simulink model "arlht_elhossini"  (R2020a)
settings: Solver=FixedStepDiscrete  StartTime=0.0  StopTime=inf  RelTol=1e-3
InitFcn:
  | % Clear workspace
  | clc; clear; close all;
  | 
  | fs = 250e6;
  | 
  | % Set parameters
  | height = 600;
  | width = 800;
  | sobelThreshold = 30;
  | dTheta = 180/16;
  | theta = (0:dTheta:180-dTheta);
  | 
  | % Derive variables
  | maxRho = ceil(sqrt((height/2)^2+(width/2)^2));
  | nRho = maxRho*2;
  | nTheta = length(theta);
  | 
  | % Read in image and resize
  | I = imread('chess.jpg');
  | Ir = imresize(I, [height, width]);
  | 
  | % Get greyscale
  | Y = rgb2gray(Ir);
  | 
  | % Get Sobel and Gradient
  | [edge, dir, mag] = SobelEdge(Y, 100);
  | dirNew = floor(dir/dTheta)*dTheta;
  | simDirNew = dirNew*4;
  | simDirNew(edge==0) = 255*4;
  | 
  | % Create input array
  | inarray = uint16(simDirNew);
StopFcn:
  | [hps, Aopt, rbm] = ARLHT(edge, dirNew, dTheta, 1, 0, 4);
  | plot3DHPS(hps);
  | 
  | simHps = reshape(out.simout, [nRho, nTheta]);
  | plot3DHPS(simHps);
values from neighbouring files (symbols this model uses):
  dir = rad2deg(atan(Gy./Gx))    [SobelEdge.m]
libraries: simulink x39, hdlsllib x26, library x3, dspsrcs4 x1
(part 1 of 2)
settings Model: DataTypeOverride=Off  SimulationMode=rapid-accelerator  Creator=david  LastModifiedBy=david
settings OptimizationCC: BlockReduction=off  ConditionallyExecuteInputs=off  DefaultParameterBehavior=Inlined
settings DebuggingCC: AlgebraicLoopMsg=error  SingleTaskRateTransMsg=error
settings HardwareCC: ProdBitPerPointer=32  ProdBitPerSizeT=32  ProdBitPerPtrDiffT=32  ProdLargestAtomicFloat=None  ProdIntDivRoundTo=Undefined  ProdEndianess=Unspecified  ProdWordSize=32  ProdHWDeviceType=ASIC/FPGA->ASIC/FPGA  TargetBitPerPointer=64  TargetBitPerSizeT=64  TargetBitPerPtrDiffT=64  TargetLongLongMode=on  TargetIntDivRoundTo=Zero  TargetEndianess=LittleEndian  TargetWordSize=64  TargetHWDeviceType=Custom Processor->MATLAB Host Computer  ProdEqTarget=off

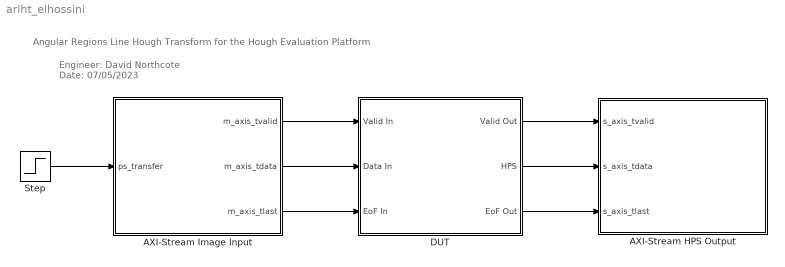
== system arlht_elhossini ==
  note: Angular Regions Line Hough Transform for the Hough Evaluation Platform
  note: Engineer: David Northcote
      | Date: 07/05/2023
  AXI-Stream HPS Output : Subsystem  mask{height=nRho, width=nTheta, clk=1/fs, d=0}
      mask prompts: height "Image Height:"; width "Image Width:"; clk "Clock Rate:"; d "Frame Capture Number"
      mask DialogControl DescGroupVar Prompt: AXI-Stream Image Output
      mask DialogControl DescTextVar Prompt: Image output using the AXI-Stream interface. Simulates an AXI DMA write channel.
      mask DialogControl ParameterGroupVar Prompt: Main
  AXI-Stream Image Input : Subsystem  mask{image=inarray, clk=1/fs}
      mask prompts: image "Input Image:"; clk "Clock Rate:"
      mask init:
      | [height, width] = size(image);
      mask DialogControl DescGroupVar Prompt: AXI-Stream Image Input
      mask DialogControl DescTextVar Prompt: This block simulates an AXI-Stream image input for interfacing to a hardware accelerator or IP Core.
      mask DialogControl ParameterGroupVar Prompt: Main
  DUT : Subsystem  TreatAsAtomicUnit=on
  Step : Step  Time=2/150e6  SampleTime=1/fs
  wires:
  AXI-Stream Image Input/1(m_axis_tvalid) -> DUT/1(Valid In)
  AXI-Stream Image Input/2(m_axis_tdata) -> DUT/2(Data In)
  AXI-Stream Image Input/3(m_axis_tlast) -> DUT/3(EoF In)
  DUT/1(Valid Out) -> AXI-Stream HPS Output/1(s_axis_tvalid)
  DUT/2(HPS) -> AXI-Stream HPS Output/2(s_axis_tdata)
  DUT/3(EoF Out) -> AXI-Stream HPS Output/3(s_axis_tlast)
  Step/1 -> AXI-Stream Image Input/1(ps_transfer)

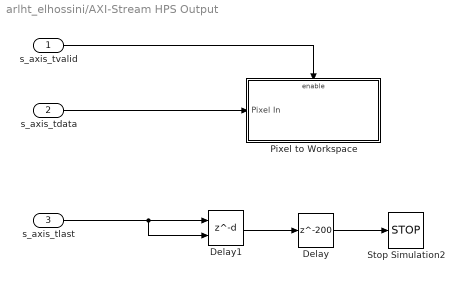
== system arlht_elhossini/AXI-Stream HPS Output ==
  s_axis_tvalid : Inport
  s_axis_tdata : Inport  Port=2
  s_axis_tlast : Inport  Port=3
  Delay : Delay  DelayLength=200
  Delay1 : Delay  DelayLength=d  ShowEnablePort=on
      settings: InputPortMap=u0,e6
  Pixel to Workspace : Subsystem
  Stop Simulation2 : Stop
  wires:
  s_axis_tvalid/1 -> Pixel to Workspace/Enable
  s_axis_tdata/1 -> Pixel to Workspace/1(Pixel In)
  s_axis_tlast/1 -> Delay1/2, Delay1/1
  Delay1/1 -> Delay/1
  Delay/1 -> Stop Simulation2/1

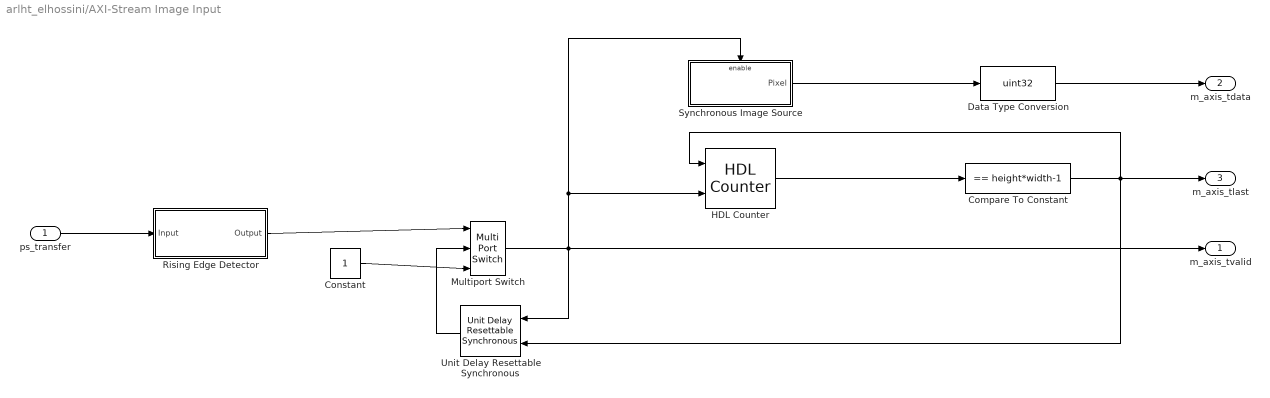
== system arlht_elhossini/AXI-Stream Image Input ==
  ps_transfer : Inport
  Compare To Constant : simulink/Logic and Bit Operations/Compare To Constant  relop===  const=height*width-1  OutDataTypeStr=boolean
  Constant : Constant  OutDataTypeStr=boolean  SampleTime=-1
  Data Type Conversion : DataTypeConversion  OutDataTypeStr=uint32
  HDL Counter : hdlsllib/Sources/HDL Counter  CountType=Free running  CountInit=0  CountStep=1  CountMax=width*height-1  CountFromType=Initial value  CountFrom=0  CountResetPort=on  CountLoadPort=off  CountEnbPort=on  CountDirPort=off  CountDataType=Unsigned  CountWordLen=32  CountFracLen=0  CountSampTime=1
  Multiport Switch : MultiPortSwitch  DataPortOrder=Zero-based contiguous  Inputs=2  zeroidx=on
  Rising Edge Detector : Subsystem
  Synchronous Image Source : Subsystem
  Unit Delay Resettable Synchronous : hdlsllib/Discrete/Unit Delay Resettable Synchronous  InitialCondition=0.0  SampleTime=-1
      settings: SourceProductBaseCode=SL
  m_axis_tvalid : Outport
  m_axis_tdata : Outport  Port=2
  m_axis_tlast : Outport  Port=3
  wires:
  HDL Counter/1 -> Compare To Constant/1
  Synchronous Image Source/1(Pixel) -> Data Type Conversion/1
  Multiport Switch/1 -> Unit Delay Resettable Synchronous/1, HDL Counter/2, Synchronous Image Source/Enable, m_axis_tvalid/1
  Compare To Constant/1 -> Unit Delay Resettable Synchronous/2, HDL Counter/1, m_axis_tlast/1
  Data Type Conversion/1 -> m_axis_tdata/1
  ps_transfer/1 -> Rising Edge Detector/1(Input)
  Unit Delay Resettable Synchronous/1 -> Multiport Switch/2
  Rising Edge Detector/1(Output) -> Multiport Switch/1
  Constant/1 -> Multiport Switch/3

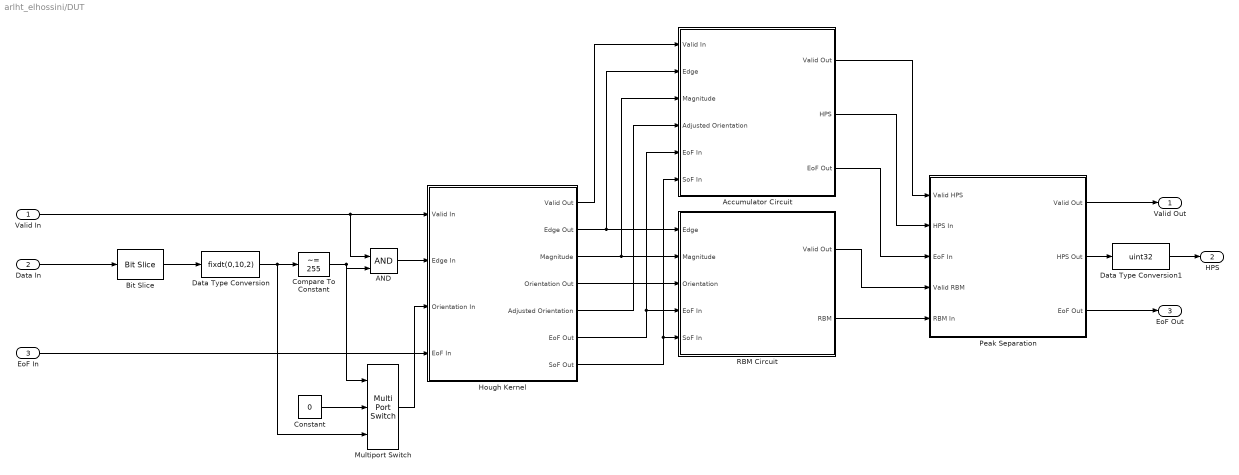
== system arlht_elhossini/DUT ==
  Valid In : Inport
  Data In : Inport  Port=2
  EoF In : Inport  Port=3
  AND : Logic  IconShape=distinctive  AllPortsSameDT=off  OutDataTypeStr=boolean
  Accumulator Circuit : Subsystem  AncestorBlock=library/Accumulator Circuit  mask{height=height, width=width, rhoBits=ceil(log2(maxRho*2*4)), nTheta=nTheta, nRho=nRho}
      mask prompts: height "Image Height:"; width "Image Width:"; rhoBits "Address Bits:"; nTheta "Number Theta:"; nRho "Number Rho:"
      mask init:
      | kTheta = 4;
  Bit Slice : hdlsllib/Logic and Bit Operations/Bit Slice  lidx=9  ridx=0
      settings: SourceProductBaseCode=SL
  Compare To Constant : simulink/Logic and Bit Operations/Compare To Constant  relop=~=  const=255  OutDataTypeStr=boolean
  Constant : Constant  Value=0  OutDataTypeStr=Inherit: Inherit via back propagation  SampleTime=-1
  Data Type Conversion : DataTypeConversion  OutDataTypeStr=fixdt(0,10,2)  ConvertRealWorld=Stored Integer (SI)
  Data Type Conversion1 : DataTypeConversion  OutDataTypeStr=uint32
  Hough Kernel : Subsystem  AncestorBlock=library/Hough Kernel  mask{rhoBits=ceil(log2(maxRho*2)), height=height, width=width, dTheta=dTheta}
      mask prompts: rhoBits "Address Bits:"; height "Image Height:"; width "Image Width:"; dTheta "Theta Resolution:"
      mask init:
      | kTheta = 4;
      | maxRho = ceil(sqrt((height/2)^2+(width/2)^2));
      | theta = (0:dTheta:180-dTheta);
      | gamma = (theta(end) + dTheta)/kTheta;
  Multiport Switch : MultiPortSwitch  DataPortOrder=Zero-based contiguous  Inputs=2  zeroidx=on
  Peak Separation : Subsystem  AncestorBlock=library/Peak Separation  mask{nRho=nRho, nTheta=nTheta}
      mask prompts: nRho "HPS Height:"; nTheta "HPS Width:"
      mask DialogControl DescGroupVar Prompt: Peak Separation
      mask DialogControl ParameterGroupVar Prompt: Main
  RBM Circuit : Subsystem  AncestorBlock=library/RBM Circuit  mask{height=height, width=width, nTheta=nTheta, rhoBits=ceil(log2(maxRho*2)), nRho=nRho}
      mask prompts: height "Image Height:"; width "Image Width:"; nTheta "Number Theta:"; rhoBits "Address Bits:"; nRho "Number Rho:"
  Valid Out : Outport  VectorParamsAs1DForOutWhenUnconnected=off
  HPS : Outport  Port=2  VectorParamsAs1DForOutWhenUnconnected=off
  EoF Out : Outport  Port=3  VectorParamsAs1DForOutWhenUnconnected=off
  wires:
  Accumulator Circuit/2(HPS) -> Peak Separation/2(HPS In)
  Hough Kernel/4(Orientation Out) -> RBM Circuit/3(Orientation)
  Hough Kernel/1(Valid Out) -> Accumulator Circuit/1(Valid In)
  Hough Kernel/3(Magnitude) -> Accumulator Circuit/3(Magnitude), RBM Circuit/2(Magnitude)
  EoF In/1 -> Hough Kernel/4(EoF In)
  RBM Circuit/2(RBM) -> Peak Separation/5(RBM In)
  Hough Kernel/5(Adjusted Orientation) -> Accumulator Circuit/4(Adjusted Orientation)
  Hough Kernel/2(Edge Out) -> Accumulator Circuit/2(Edge), RBM Circuit/1(Edge)
  Hough Kernel/6(EoF Out) -> Accumulator Circuit/5(EoF In), RBM Circuit/4(EoF In)
  Hough Kernel/7(SoF Out) -> Accumulator Circuit/6(SoF In), RBM Circuit/5(SoF In)
  Peak Separation/2(HPS Out) -> Data Type Conversion1/1
  Peak Separation/3(EoF Out) -> EoF Out/1
  RBM Circuit/1(Valid Out) -> Peak Separation/4(Valid RBM)
  Peak Separation/1(Valid Out) -> Valid Out/1
  Accumulator Circuit/1(Valid Out) -> Peak Separation/1(Valid HPS)
  Accumulator Circuit/3(EoF Out) -> Peak Separation/3(EoF In)
  Multiport Switch/1 -> Hough Kernel/3(Orientation In)
  Constant/1 -> Multiport Switch/2
  Data In/1 -> Bit Slice/1
  Data Type Conversion/1 -> Multiport Switch/3, Compare To Constant/1
  AND/1 -> Hough Kernel/2(Edge In)
  Compare To Constant/1 -> AND/2, Multiport Switch/1
  Valid In/1 -> AND/1, Hough Kernel/1(Valid In)
  Data Type Conversion1/1 -> HPS/1
  Bit Slice/1 -> Data Type Conversion/1

== system arlht_elhossini/AXI-Stream HPS Output/Pixel to Workspace ==
  Pixel In : Inport
  Enable : EnablePort
  To Workspace : ToWorkspace  VariableName=simout  SampleTime=-1
      settings: MaxDataPoints=height*width  Save2DSignal=2-D array (concatenate along first dimension)
  wires:
  Pixel In/1 -> To Workspace/1

== system arlht_elhossini/AXI-Stream Image Input/Rising Edge Detector ==
  Input : Inport
  AND : Logic  IconShape=distinctive  AllPortsSameDT=off  OutDataTypeStr=boolean
  Delay : Delay  DelayLength=1
  NOT : Logic  Operator=NOT  IconShape=distinctive  AllPortsSameDT=off  OutDataTypeStr=boolean
  Output : Outport  VectorParamsAs1DForOutWhenUnconnected=off
  wires:
  NOT/1 -> Delay/1
  Input/1 -> AND/2, NOT/1
  Delay/1 -> AND/1
  AND/1 -> Output/1

== system arlht_elhossini/AXI-Stream Image Input/Synchronous Image Source ==
  Enable : EnablePort
  Signal From Workspace : dspsrcs4/Signal From Workspace  X=reshape(image', [height*width, 1])  Ts=clk  nsamps=1  OutputAfterFinalValue=Cyclic repetition  ignoreOrWarnInputAndFrameLengths=off  OutputFrames=off
  Pixel : Outport
  wires:
  Signal From Workspace/1 -> Pixel/1

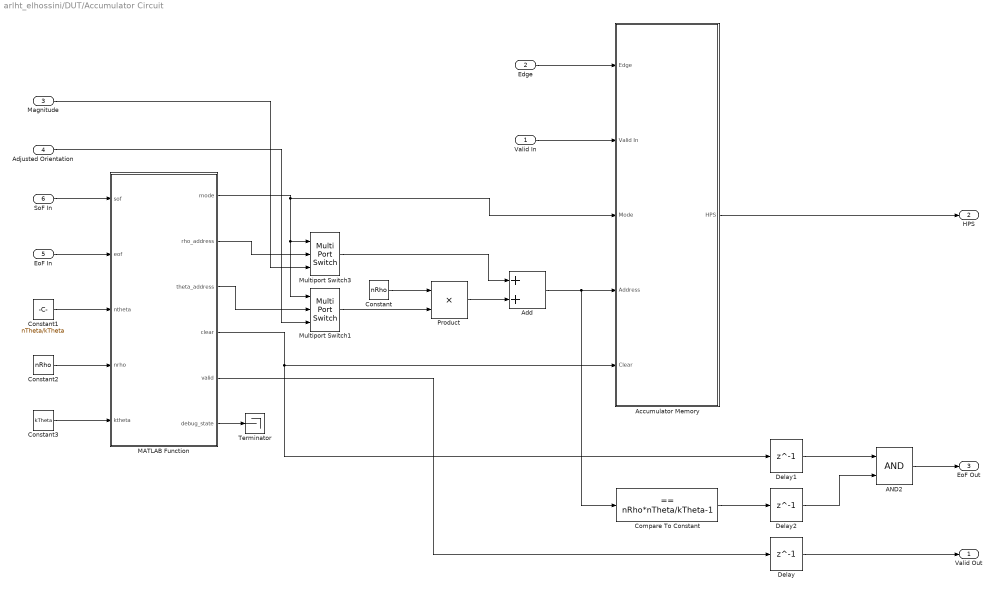
== system arlht_elhossini/DUT/Accumulator Circuit ==
  Valid In : Inport
  Edge : Inport  Port=2
  Magnitude : Inport  Port=3
  Adjusted Orientation : Inport  Port=4
  EoF In : Inport  Port=5
  SoF In : Inport  Port=6
  AND2 : Logic  IconShape=distinctive  AllPortsSameDT=off  OutDataTypeStr=boolean
  Accumulator Memory : Subsystem
  Add : Sum  OutDataTypeStr=fixdt(0,ceil(log2(nRho*nTheta/kTheta)),0)
  Compare To Constant : simulink/Logic and Bit Operations/Compare To Constant  relop===  const=nRho*nTheta/kTheta-1  OutDataTypeStr=boolean
  Constant : Constant  Value=nRho  OutDataTypeStr=fixdt(0,ceil(log2(nRho+1)),0)  SampleTime=-1
  Constant1 : Constant  Value=nTheta/kTheta  OutDataTypeStr=uint8  SampleTime=-1
  Constant2 : Constant  Value=nRho  OutDataTypeStr=uint16  SampleTime=-1
  Constant3 : Constant  Value=kTheta  OutDataTypeStr=uint8  SampleTime=-1
  Delay : Delay  DelayLength=1  InitialCondition=0  UseCircularBuffer=on
  Delay1 : Delay  DelayLength=1  InitialCondition=0  UseCircularBuffer=on
  Delay2 : Delay  DelayLength=1  InitialCondition=0  UseCircularBuffer=on
  MATLAB Function : MATLAB Function  TreatAsAtomicUnit=on
  Multiport Switch1 : MultiPortSwitch  DataPortOrder=Zero-based contiguous  Inputs=2  zeroidx=on
  Multiport Switch3 : MultiPortSwitch  DataPortOrder=Zero-based contiguous  Inputs=2  zeroidx=on
  Product : Product  OutDataTypeStr=fixdt(0,ceil(log2(nRho*(nTheta/kTheta-1))),0)
  Terminator : Terminator
  Valid Out : Outport
  HPS : Outport  Port=2
  EoF Out : Outport  Port=3
  wires:
  MATLAB Function/6(debug_state) -> Terminator/1
  SoF In/1 -> MATLAB Function/1(sof)
  MATLAB Function/4(clear) -> Delay1/1, Accumulator Memory/5(Clear)
  MATLAB Function/5(valid) -> Delay/1
  Delay/1 -> Valid Out/1
  AND2/1 -> EoF Out/1
  Delay1/1 -> AND2/1
  Delay2/1 -> AND2/2
  Constant1/1 -> MATLAB Function/3(ntheta)
  Constant2/1 -> MATLAB Function/4(nrho)
  Constant3/1 -> MATLAB Function/5(ktheta)
  Compare To Constant/1 -> Delay2/1
  Magnitude/1 -> Multiport Switch3/3
  Adjusted Orientation/1 -> Multiport Switch1/3
  Edge/1 -> Accumulator Memory/1(Edge)
  Valid In/1 -> Accumulator Memory/2(Valid In)
  Accumulator Memory/1(HPS) -> HPS/1
  Add/1 -> Compare To Constant/1, Accumulator Memory/4(Address)
  Multiport Switch1/1 -> Product/2
  Multiport Switch3/1 -> Add/1
  Product/1 -> Add/2
  Constant/1 -> Product/1
  MATLAB Function/1(mode) -> Multiport Switch1/1, Multiport Switch3/1, Accumulator Memory/3(Mode)
  MATLAB Function/2(rho_address) -> Multiport Switch3/2
  MATLAB Function/3(theta_address) -> Multiport Switch1/2
  EoF In/1 -> MATLAB Function/2(eof)

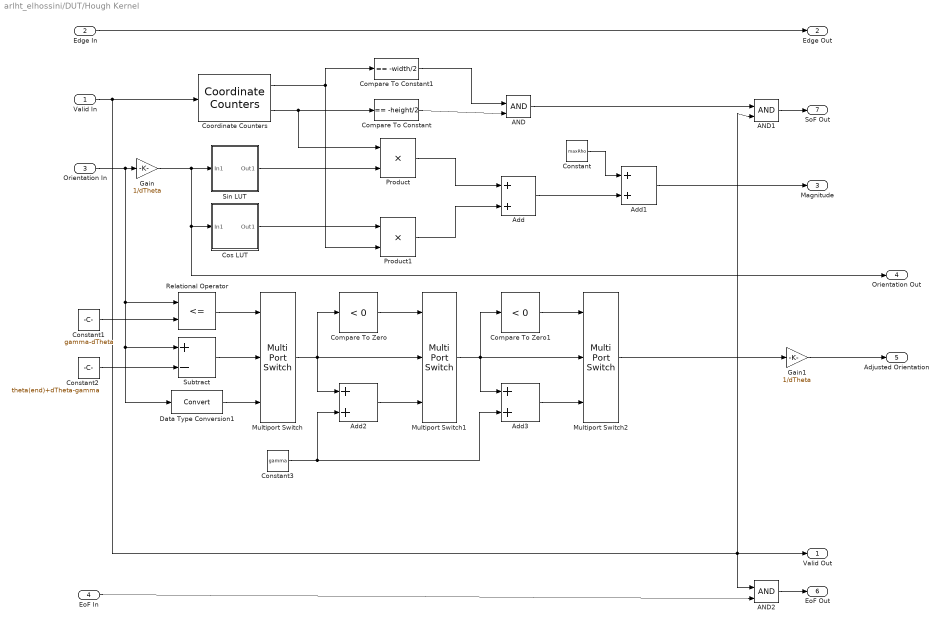
== system arlht_elhossini/DUT/Hough Kernel ==
  Valid In : Inport
  Edge In : Inport  Port=2
  Orientation In : Inport  Port=3
  EoF In : Inport  Port=4
  AND : Logic  IconShape=distinctive  AllPortsSameDT=off  OutDataTypeStr=boolean
  AND1 : Logic  IconShape=distinctive  AllPortsSameDT=off  OutDataTypeStr=boolean
  AND2 : Logic  IconShape=distinctive  AllPortsSameDT=off  OutDataTypeStr=boolean
  Add : Sum
  Add1 : Sum  OutDataTypeStr=fixdt(0,rhoBits,0)
  Add2 : Sum  OutDataTypeStr=Inherit: Same as first input
  Add3 : Sum  OutDataTypeStr=Inherit: Same as first input
  Compare To Constant : simulink/Logic and Bit Operations/Compare To Constant  relop===  const=-height/2  OutDataTypeStr=boolean
  Compare To Constant1 : simulink/Logic and Bit Operations/Compare To Constant  relop===  const=-width/2  OutDataTypeStr=boolean
  Compare To Zero : simulink/Logic and Bit Operations/Compare To Zero  relop=<  OutDataTypeStr=boolean
  Compare To Zero1 : simulink/Logic and Bit Operations/Compare To Zero  relop=<  OutDataTypeStr=boolean
  Constant : Constant  Value=maxRho  OutDataTypeStr=fixdt(0,ceil(log2(maxRho+1)),0)  SampleTime=-1
  Constant1 : Constant  Value=gamma-dTheta  OutDataTypeStr=fixdt(0,ceil(log2(gamma))+2,2)  SampleTime=-1
  Constant2 : Constant  Value=theta(end)+dTheta-gamma  OutDataTypeStr=fixdt(0,ceil(log2(179+1-gamma))+2,2)  SampleTime=-1
  Constant3 : Constant  Value=gamma  OutDataTypeStr=fixdt(0,ceil(log2(gamma+1)),0)  SampleTime=-1
  Coordinate Counters : library/Coordinate Counters  height=height  width=width
  Cos LUT : Subsystem
  Data Type Conversion1 : DataTypeConversion
  Gain : Gain  Gain=1/dTheta  ParamDataTypeStr=fixdt(0,20,20)  OutDataTypeStr=fixdt(0,ceil(log2(nTheta)),0)  SaturateOnIntegerOverflow=on
  Gain1 : Gain  Gain=1/dTheta  ParamDataTypeStr=fixdt(0,20,20)  OutDataTypeStr=fixdt(0,ceil(log2(nTheta)),0)  SaturateOnIntegerOverflow=on
  Multiport Switch : MultiPortSwitch  DataPortOrder=Zero-based contiguous  Inputs=2  zeroidx=on
  Multiport Switch1 : MultiPortSwitch  DataPortOrder=Zero-based contiguous  Inputs=2  zeroidx=on
  Multiport Switch2 : MultiPortSwitch  DataPortOrder=Zero-based contiguous  Inputs=2  zeroidx=on
  Product : Product  OutDataTypeStr=fixdt(1,ceil(log2(height)),0)  RndMeth=Round
  Product1 : Product  OutDataTypeStr=fixdt(1,ceil(log2(width)),0)  RndMeth=Round
  Relational Operator : RelationalOperator  Operator=<=  OutDataTypeStr=boolean  RndMeth=Simplest
  Sin LUT : Subsystem
  Subtract : Sum  Inputs=+-  OutDataTypeStr=fixdt(1,10,2)
  Valid Out : Outport
  Edge Out : Outport  Port=2
  Magnitude : Outport  Port=3
  Orientation Out : Outport  Port=4
  Adjusted Orientation : Outport  Port=5
  EoF Out : Outport  Port=6
  SoF Out : Outport  Port=7
  wires:
  Sin LUT/1(Out1) -> Product/2
  Cos LUT/1(Out1) -> Product1/1
  EoF In/1 -> AND2/2
  AND2/1 -> EoF Out/1
  Valid In/1 -> Coordinate Counters/1, Valid Out/1, AND1/2, AND2/1
  AND/1 -> AND1/1
  AND1/1 -> SoF Out/1
  Compare To Constant/1 -> AND/2
  Compare To Constant1/1 -> AND/1
  Constant1/1 -> Relational Operator/2
  Orientation In/1 -> Data Type Conversion1/1, Subtract/1, Relational Operator/1, Gain/1
  Compare To Zero/1 -> Multiport Switch1/1
  Multiport Switch1/1 -> Multiport Switch2/2, Compare To Zero1/1, Add3/1
  Multiport Switch/1 -> Multiport Switch1/2, Compare To Zero/1, Add2/1
  Compare To Zero1/1 -> Multiport Switch2/1
  Product/1 -> Add/1
  Subtract/1 -> Multiport Switch/2
  Add1/1 -> Magnitude/1
  Add2/1 -> Multiport Switch1/3
  Add3/1 -> Multiport Switch2/3
  Constant2/1 -> Subtract/2
  Constant3/1 -> Add2/2, Add3/2
  Add/1 -> Add1/2
  Relational Operator/1 -> Multiport Switch/1
  Constant/1 -> Add1/1
  Product1/1 -> Add/2
  Coordinate Counters/1 -> Compare To Constant1/1, Product1/2
  Coordinate Counters/2 -> Compare To Constant/1, Product/1
  Edge In/1 -> Edge Out/1
  Multiport Switch2/1 -> Gain1/1
  Gain/1 -> Orientation Out/1, Cos LUT/1(In1), Sin LUT/1(In1)
  Gain1/1 -> Adjusted Orientation/1
  Data Type Conversion1/1 -> Multiport Switch/3

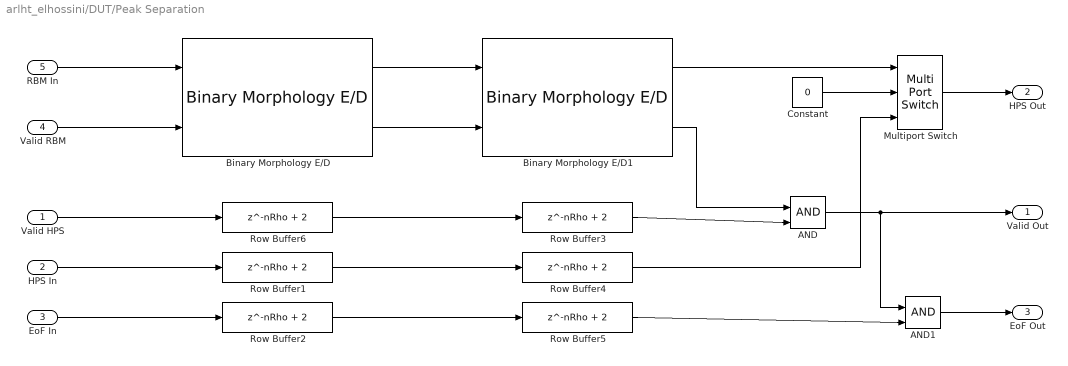
== system arlht_elhossini/DUT/Peak Separation ==
  Valid HPS : Inport
  HPS In : Inport  Port=2
  EoF In : Inport  Port=3
  Valid RBM : Inport  Port=4
  RBM In : Inport  Port=5
  AND : Logic  IconShape=distinctive  AllPortsSameDT=off  OutDataTypeStr=boolean
  AND1 : Logic  IconShape=distinctive  AllPortsSameDT=off  OutDataTypeStr=boolean
  Binary Morphology E/D : library/Binary Morphology E//D  operation=Erosion  height=nTheta  width=nRho
  Binary Morphology E/D1 : library/Binary Morphology E//D  operation=Dilation  height=nTheta  width=nRho
  Constant : Constant  Value=0  OutDataTypeStr=Inherit: Inherit via back propagation  SampleTime=-1
  Multiport Switch : MultiPortSwitch  DataPortOrder=Zero-based contiguous  Inputs=2  zeroidx=on
  Row Buffer{1..6} (6 alike) : Delay  DelayLength=nRho + 2
  Valid Out : Outport
  HPS Out : Outport  Port=2
  EoF Out : Outport  Port=3
  wires:
  Row Buffer5/1 -> AND1/2
  AND/1 -> Valid Out/1, AND1/1
  Row Buffer4/1 -> Multiport Switch/3
  Binary Morphology E/D/2 -> Binary Morphology E/D1/2
  Binary Morphology E/D/1 -> Binary Morphology E/D1/1
  Valid RBM/1 -> Binary Morphology E/D/2
  RBM In/1 -> Binary Morphology E/D/1
  EoF In/1 -> Row Buffer2/1
  HPS In/1 -> Row Buffer1/1
  Valid HPS/1 -> Row Buffer6/1
  Binary Morphology E/D1/2 -> AND/1
  Row Buffer3/1 -> AND/2
  Constant/1 -> Multiport Switch/2
  Row Buffer1/1 -> Row Buffer4/1
  Row Buffer6/1 -> Row Buffer3/1
  Binary Morphology E/D1/1 -> Multiport Switch/1
  Row Buffer2/1 -> Row Buffer5/1
  AND1/1 -> EoF Out/1
  Multiport Switch/1 -> HPS Out/1

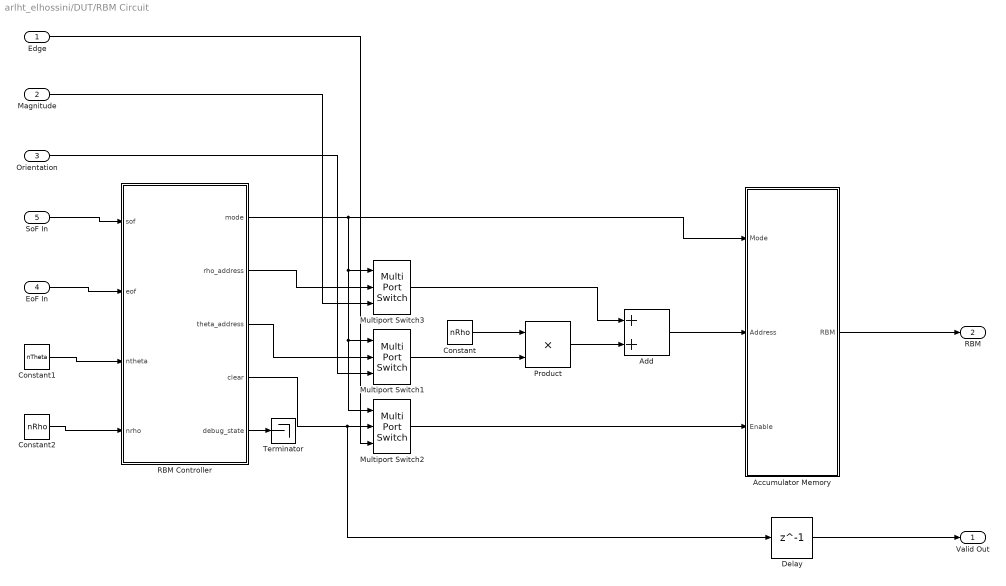
== system arlht_elhossini/DUT/RBM Circuit ==
  Edge : Inport
  Magnitude : Inport  Port=2
  Orientation : Inport  Port=3
  EoF In : Inport  Port=4
  SoF In : Inport  Port=5
  Accumulator Memory : Subsystem
  Add : Sum  OutDataTypeStr=fixdt(0,ceil(log2(nRho*nTheta)),0)
  Constant : Constant  Value=nRho  OutDataTypeStr=fixdt(0,ceil(log2(nRho+1)),0)  SampleTime=-1
  Constant1 : Constant  Value=nTheta  OutDataTypeStr=uint8  SampleTime=-1
  Constant2 : Constant  Value=nRho  OutDataTypeStr=uint16  SampleTime=-1
  Delay : Delay  DelayLength=1  InitialCondition=0  UseCircularBuffer=on
  Multiport Switch1 : MultiPortSwitch  DataPortOrder=Zero-based contiguous  Inputs=2  zeroidx=on
  Multiport Switch2 : MultiPortSwitch  DataPortOrder=Zero-based contiguous  Inputs=2  zeroidx=on
  Multiport Switch3 : MultiPortSwitch  DataPortOrder=Zero-based contiguous  Inputs=2  zeroidx=on
  Product : Product  OutDataTypeStr=fixdt(0,ceil(log2(nRho*(nTheta))),0)
  RBM Controller : MATLAB Function  TreatAsAtomicUnit=on
  Terminator : Terminator
  Valid Out : Outport
  RBM : Outport  Port=2
  wires:
  RBM Controller/5(debug_state) -> Terminator/1
  RBM Controller/3(theta_address) -> Multiport Switch1/2
  RBM Controller/2(rho_address) -> Multiport Switch3/2
  RBM Controller/1(mode) -> Multiport Switch3/1, Multiport Switch2/1, Multiport Switch1/1, Accumulator Memory/1(Mode)
  Constant/1 -> Product/1
  Product/1 -> Add/2
  Multiport Switch3/1 -> Add/1
  Multiport Switch1/1 -> Product/2
  Add/1 -> Accumulator Memory/2(Address)
  Accumulator Memory/1(RBM) -> RBM/1
  Orientation/1 -> Multiport Switch1/3
  Magnitude/1 -> Multiport Switch3/3
  Constant2/1 -> RBM Controller/4(nrho)
  Constant1/1 -> RBM Controller/3(ntheta)
  Delay/1 -> Valid Out/1
  RBM Controller/4(clear) -> Multiport Switch2/2, Delay/1
  SoF In/1 -> RBM Controller/1(sof)
  Edge/1 -> Multiport Switch2/3
  Multiport Switch2/1 -> Accumulator Memory/3(Enable)
  EoF In/1 -> RBM Controller/2(eof)

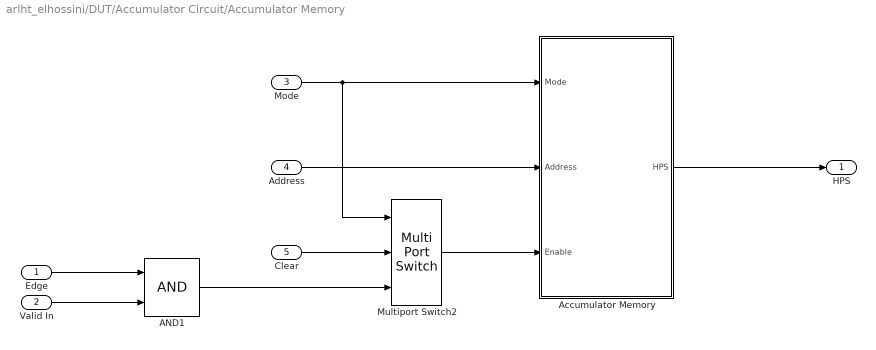
== system arlht_elhossini/DUT/Accumulator Circuit/Accumulator Memory ==
  Edge : Inport
  Valid In : Inport  Port=2
  Mode : Inport  Port=3
  Address : Inport  Port=4
  Clear : Inport  Port=5
  AND1 : Logic  IconShape=distinctive  AllPortsSameDT=off  OutDataTypeStr=boolean
  Accumulator Memory : Subsystem
  Multiport Switch2 : MultiPortSwitch  DataPortOrder=Zero-based contiguous  Inputs=2  zeroidx=on
  HPS : Outport
  wires:
  Mode/1 -> Multiport Switch2/1, Accumulator Memory/1(Mode)
  Multiport Switch2/1 -> Accumulator Memory/3(Enable)
  Address/1 -> Accumulator Memory/2(Address)
  Valid In/1 -> AND1/2
  Accumulator Memory/1(HPS) -> HPS/1
  AND1/1 -> Multiport Switch2/3
  Edge/1 -> AND1/1
  Clear/1 -> Multiport Switch2/2

== system arlht_elhossini/DUT/Hough Kernel/Cos LUT ==
  In1 : Inport
  1-D Lookup Table : Lookup_n-D  NumberOfTableDimensions=1  BreakpointsForDimension1=(0:1:length(theta)-1)  IndexSearchMethod=Evenly spaced points  Table=cos(deg2rad(theta))  InterpMethod=Flat  DiagnosticForOutOfRangeInput=Error  InternalRulePriority=Speed  OutDataTypeStr=fixdt(1,16,14)  RndMeth=Simplest  InputSameDT=on
  Out1 : Outport
  wires:
  1-D Lookup Table/1 -> Out1/1
  In1/1 -> 1-D Lookup Table/1

== system arlht_elhossini/DUT/Hough Kernel/Sin LUT ==
  In1 : Inport
  1-D Lookup Table : Lookup_n-D  NumberOfTableDimensions=1  BreakpointsForDimension1=(0:1:length(theta)-1)  IndexSearchMethod=Evenly spaced points  Table=sin(deg2rad(theta))  InterpMethod=Flat  DiagnosticForOutOfRangeInput=Error  InternalRulePriority=Speed  OutDataTypeStr=fixdt(1,16,14)  RndMeth=Simplest  InputSameDT=on
  Out1 : Outport
  wires:
  In1/1 -> 1-D Lookup Table/1
  1-D Lookup Table/1 -> Out1/1

== system arlht_elhossini/DUT/RBM Circuit/Accumulator Memory ==
  Mode : Inport
  Address : Inport  Port=2
  Enable : Inport  Port=3
  simple_block_ram : Subsystem  VariantControl=other_bits  mask{b=1, d=nRho*nTheta, b_hidden=36, d_hidden=98304}
      mask prompts: b "Data width:"; d "Depth:"
      mask init:
      | if d == d_hidden
      |     return
      | end
      | 
      | set_param(gcb, 'd_hidden', int2str(d));
      | 
      | % Xilinx RAM Initialisation
      | xl_config = [512, 72;
      |             1024, 36;
      |             2048, 18;
      |             4096, 9;
      |             8192, 4;
      |             16384, 2;
      |             32768, 1];
      | 
      | % Get length of Xilinx Configuration
      | sizeram = size(xl_config);
      |         
      | % Get the RAM Configuration based on the data width
      | for i = 1:sizeram(1)
      |     if b <= xl_config(i, 2)
      |         a = xl_config(i, :);
      |     end
      | end
      | 
      | % Get number of BRAM required (including half BRAM)
      | numbram = ceil((d/a(1))/0.5)*0.5;
      | fullbram = floor(numbram); % Integer
      | halfbram = (numbram-floor(numbram)) ~= 0; % Boolean
      | 
      | % Get all blocks and delete everything excepts ports
      | H = get(find_system(gcb, 'FindAll', 'on', 'type', 'block'));
      | todelete = setdiff(strcat(repmat({[gcb '/']}, numel(H.Blocks), 1),  H.Blocks),...
      |     strcat(repmat({[gcb '/']}, 5, 1),...
      |     {'wr_data'; 'wr_addr'; 'wr_en'; 'rd_addr'; 'rd_data'}));
      | delete_block(todelete);
      | 
      | % Delete lines
      | for i = 1:numel(H.Lines)
      |     delete_line(H.Lines(i).Handle)
      | end
      | 
      | % Generate full BRAMs
      | y = 0;
      | 
      | % If there is only one ram then the write enable should be directly
      | % connected to the first ram write enable. Else, the write address must be sliced
      | % and the upper bound (over a(2)) compared to zero. This will indicate if
      | % the first ram is the one to be written/read from.
      | 
      | % Common to both implementations
      | % Write Address Slice
      | add_block('hdlsllib/Logic and Bit Operations/Bit Slice',...
      |         [gcb, '/wr_address'], 'Position',...
      |         [160 130 250 170]);
      | % Set bitslice parameters
      | set_param([gcb, '/wr_address'],...
      |     'lidx', int2str(log2(a(1))-1));
      | set_param([gcb, '/wr_address'],...
      |     'ridx', int2str(0));
      | 
      | % Read Address Slice
      | add_block('hdlsllib/Logic and Bit Operations/Bit Slice',...
      |         [gcb, '/rd_address'], 'Position',...
      |         [160 330 250 370]);
      | % Set bitslice parameters
      | set_param([gcb, '/rd_address'],...
      |     'lidx', int2str(log2(a(1))-1));
      | set_param([gcb, '/rd_address'],...
      |     'ridx', int2str(0));
      | 
      | if ceil(numbram) == 1
      |     
      |     i = 1;
      |     
      |     % Set bitslice parameters
      |     set_param([gcb, '/rd_address'],...
      |         'lidx', int2str(ceil(log2(d))-1));
      |     set_param([gcb, '/wr_address'],...
      |         'lidx', int2str(ceil(log2(d))-1));
      |     
      |     % Add Simple RAM
      |     add_block('hdlsllib/HDL RAMs/Simple Dual Port RAM',...
      |         [gcb, '/simple_ram_', int2str(i-1)], 'Position',...
      |         [635 0+600*y 635+200 400+600*y]);
      | 
      |     % Set RAM parameters
      |     set_param([gcb, '/simple_ram_', int2str(i-1)],...
      |         'ram_size', int2str(ceil(log2(d))));
      | 
      |     % Connect "wr_data" to "simple_ram_i"
      |     add_line(gcb, ['wr_data/1'], ['simple_ram_', int2str(i-1), '/1'],...
      |         'autorouting', 'on');
      |     
      |     % Connect "wr_addr" to "wr_address"
      |     add_line(gcb, ['wr_addr/1'], ['wr_address/1'],...
      |         'autorouting', 'on');
      | 
      |     % Connect "wr_address" to "simple_ram_i"
      |     add_line(gcb, ['wr_address/1'], ['simple_ram_', int2str(i-1), '/2'],...
      |         'autorouting', 'on');
      | 
      |     % Connect "wr_en" to "simple_ram_i"
      |     add_line(gcb, ['wr_en/1'], ['simple_ram_', int2str(i-1), '/3'],...
      |         'autorouting', 'on');
      |     
      |     % Connect "rd_addr" to "rd_address"
      |     add_line(gcb, ['rd_addr/1'], ['rd_address/1'],...
      |         'autorouting', 'on');
      | 
      |     % Connect "rd_address" to "simple_ram_i"
      |     add_line(gcb, ['rd_address/1'], ['simple_ram_', int2str(i-1), '/4'],...
      |         'autorouting', 'on');
      |     
      |     % Connect "simple_ram_i" to "rd_data"
      |     add_line(gcb, ['simple_ram_', int2str(i-1), '/1'], ['rd_data/1'],...
      |         'autorouting', 'on');
      | 
      | else
      |     
      |     % Multiport Switch
      |     add_block('hdlsllib/Signal Routing/Multiport Switch',...
      |         [gcb, '/multiport_switch'], 'Position',...
      |         [1340 146 1405 250]);
      |     % Set multiport switch parameters
      |     set_param([gcb, '/multiport_switch'],...
      |         'Inputs', int2str(ceil(numbram)));
      |     set_param([gcb, '/multiport_switch'],...
      |         'DataPortOrder', 'Zero-based contiguous');
      | 
      |     % Add Constant Zero
      |     add_block('hdlsllib/Sources/Constant',...
      |         [gcb, '/zero'], 'Position',...
      |         [425 -65 455 -35]);
      |     set_param([gcb, '/zero'],...
      |         'Value', int2str(0));
      |     set_param([gcb, '/zero'],...
      |         'OutDataTypeStr', ['fixdt(0, ', int2str(ceil(numbram)), ', 0)']);
      | 
      |     % Add Vector Concatenate
      |     add_block('hdlsllib/Signal Routing/Vector Concatenate',...
      |         [gcb, '/vector_concatenate'], 'Position',...
      |         [1015, -113, 1025, 38]);
      |     set_param([gcb, '/vector_concatenate'],...
      |         'NumInputs', int2str(ceil(numbram)));
      | 
      |     % Add Bitwise-OR
      |     add_block('hdlsllib/Logic and Bit Operations/Bitwise Operator',...
      |         [gcb, '/bitwise_or'], 'Position',...
      |         [1165, -54, 1205, -16]);
      |     set_param([gcb, '/bitwise_or'],...
      |         'logicop', 'OR');
      |     set_param([gcb, '/bitwise_or'],...
      |         'UseBitMask', 0);
      |     set_param([gcb, '/bitwise_or'],...
      |         'NumInputPorts', int2str(1));
      | 
      |     % Add delay for bram access
      |     add_block('hdlsllib/Discrete/Delay',...
      |         [gcb, '/delay'], 'Position',...
      |         [1248, 60, 1282, 95]);
      |     set_param([gcb, '/delay'],...
      |         'DelayLength', int2str(1));
      |     
      |     % Add bitslice
      |     add_block('hdlsllib/Logic and Bit Operations/Bit Slice',...
      |         [gcb, '/wr_bitslice'], 'Position',...
      |         [-65 180 25 220]);
      | 
      |     % Set bitslice parameters
      |     set_param([gcb, '/wr_bitslice'],...
      |         'lidx', int2str(ceil(log2(d)-1)));
      |     set_param([gcb, '/wr_bitslice'],...
      |         'ridx', int2str(log2(a(1))));
      |     
      |     % Add bitslice
      |     add_block('hdlsllib/Logic and Bit Operations/Bit Slice',...
      |         [gcb, '/rd_bitslice'], 'Position',...
      |         [-65 280 25 320]);
      | 
      |     % Set bitslice parameters
      |     set_param([gcb, '/rd_bitslice'],...
      |         'lidx', int2str(ceil(log2(d)-1)));
      |     set_param([gcb, '/rd_bitslice'],...
      |         'ridx', int2str(log2(a(1))));
      |     
      |     for i = 1:ceil(numbram)
      |         
      |         %%%%% Begin Adding Blocks %%%%%
      |         % Add Simple RAM
      |         add_block('hdlsllib/HDL RAMs/Simple Dual Port RAM',...
      |             [gcb, '/simple_ram_', int2str(i-1)], 'Position',...
      |             [635 0+600*y 635+200 400+600*y]);
      | 
      |         % Set RAM parameters
      |         set_param([gcb, '/simple_ram_', int2str(i-1)],...
      |             'ram_size', int2str(log2(a(1))));
      | 
      |         % Add compare to constant
      |         add_block('hdlsllib/Logic and Bit Operations/Compare To Constant',...
      |             [gcb, '/wr_cmp2const_', int2str(i-1)], 'Position',...
      |             [190 225+y*600 220 255+y*600]); 
      | 
      |         % Set compare to zero parameters
      |         set_param([gcb, '/wr_cmp2const_', int2str(i-1)],...
      |             'relop', '==');
      | 
      |         % Set compare to zero parameters
      |         set_param([gcb, '/wr_cmp2const_', int2str(i-1)],...
      |             'const', int2str(i-1));
      |         
      |         % Add compare to constant
      |         add_block('hdlsllib/Logic and Bit Operations/Compare To Constant',...
      |             [gcb, '/rd_cmp2const_', int2str(i-1)], 'Position',...
      |             [190 445+y*600 220 475+y*600]); 
      | 
      |         % Set compare to zero parameters
      |         set_param([gcb, '/rd_cmp2const_', int2str(i-1)],...
      |             'relop', '==');
      | 
      |         % Set compare to zero parameters
      |         set_param([gcb, '/rd_cmp2const_', int2str(i-1)],...
      |             'const', int2str(i-1));
      | 
      |         % Add and logic
      |         add_block('hdlsllib/Logic and Bit Operations/Logical Operator',...
      |             [gcb, '/and_', int2str(i-1)], 'Position',...
      |             [420 231+600*y 455 264+600*y]);
      | 
      |         % Set and logic parameters
      |         set_param([gcb, '/and_', int2str(i-1)],...
      |             'Operator', 'AND');
      | 
      |         % Add Switch
      |         add_block('hdlsllib/Signal Routing/Switch',...
      |             [gcb, '/switch_', int2str(i-1)], 'Position',...
      |             [685 -113+600*y 785 -37+600*y]);
      | 
      |         % Set switch parameters
      |         set_param([gcb, '/switch_', int2str(i-1)],...
      |             'Threshold', int2str(1));
      | 
      |         % Add Constant
      |         add_block('hdlsllib/Sources/Constant',...
      |             [gcb, '/constant_', int2str(i-1)], 'Position',...
      |             [425 -115+600*y 455 -85+600*y]);
      | 
      |         % Set Constant parameters
      |         set_param([gcb, '/constant_', int2str(i-1)],...
      |             'Value', int2str(i-1));
      |         set_param([gcb, '/constant_', int2str(i-1)],...
      |             'OutDataTypeStr', ['fixdt(0, ', int2str(ceil(numbram)), ', 0)']);   
      | 
      |         %%%%% Begin Wire Connections %%%%%        
      |         % Connect "wr_data" to "simple_ram_i"
      |         add_line(gcb, 'wr_data/1', ['simple_ram_', int2str(i-1), '/1'],...
      |             'autorouting','on');
      | 
      |         % Connect "wr_address" to "simple_ram_i"
      |         add_line(gcb, 'wr_address/1', ['simple_ram_', int2str(i-1), '/2'],...
      |             'autorouting','on');
      | 
      |         % Connect "rd_address" to "simple_ram_i"
      |         add_line(gcb, 'rd_address/1', ['simple_ram_', int2str(i-1), '/4'],...
      |             'autorouting','on');
      | 
      |         % Connect "constant_i" to "switch_i"
      |         add_line(gcb, ['constant_', int2str(i-1), '/1'], ['switch_', int2str(i-1), '/1'],...
      |             'autorouting','on');
      | 
      |         % Connect "zero" to "switch_i"
      |         add_line(gcb, 'zero/1', ['switch_', int2str(i-1), '/3'],...
      |             'autorouting','on');
      | 
      |         % Connect "switch_i" to "vector_concatenate"
      |         add_line(gcb, ['switch_', int2str(i-1), '/1'], ['vector_concatenate/', int2str(i)],...
      |             'autorouting','on');
      | 
      |         % Connect "rd_address" to "simple_ram_i"
      |         add_line(gcb, ['simple_ram_', int2str(i-1), '/1'], ['multiport_switch/', int2str(i+1)],...
      |             'autorouting','on');
      | 
      |         % Connect "bitslice_i" to "wr_cmp2const_i"
      |         add_line(gcb, ['wr_bitslice/1'], ['wr_cmp2const_', int2str(i-1), '/1'],...
      |             'autorouting','on');
      |         
      |         % Connect "bitslice_i" to "rd_cmp2const_i"
      |         add_line(gcb, ['rd_bitslice/1'], ['rd_cmp2const_', int2str(i-1), '/1'],...
      |             'autorouting','on');
      | 
      |         % Connect "wr_en" to "and_i"
      |         add_line(gcb, ['wr_en/1'], ['and_', int2str(i-1), '/2'],...
      |             'autorouting','on');
      | 
      |         % Connect "and_i" to "simple_ram_0"
      |         add_line(gcb, ['and_', int2str(i-1), '/1'], ['simple_ram_', int2str(i-1), '/3'],...
      |             'autorouting','on');
      | 
      |         % Connect "wr_cmp2const_i" to "and_i"
      |         add_line(gcb, ['wr_cmp2const_', int2str(i-1), '/1'], ['and_', int2str(i-1), '/1'],...
      |             'autorouting','on');
      | 
      |         % Connect "rd_cmp2const_i" to "switch_i"
      |         add_line(gcb, ['rd_cmp2const_', int2str(i-1), '/1'], ['switch_', int2str(i-1), '/2'],...
      |             'autorouting','on');
      |          
      |         % Update coordinates
      |         y = y + 1;
      |         
      |     end
      |     
      |     % Connect "rd_addr" to "bitslice_i"
      |     add_line(gcb, ['rd_addr/1'], ['rd_bitslice/1'],...
      |         'autorouting','on');
      |     
      |     % Connect "wr_addr" to "bitslice_i"
      |     add_line(gcb, ['wr_addr/1'], ['wr_bitslice/1'],...
      |         'autorouting','on');
      |     
      |     % Connect "wr_addr" to "wr_address"
      |     add_line(gcb, 'wr_addr/1', ['wr_address', '/1'],...
      |         'autorouting','on');
      | 
      |     % Connect "rd_addr" to "rd_address"
      |     add_line(gcb, 'rd_addr/1', ['rd_address', '/1'],...
      |         'autorouting','on');
      | 
      |     % Connect "vector_concatenate" to "bitwise_or"
      |     add_line(gcb, ['vector_concatenate/1'], ['bitwise_or/1'],...
      |         'autorouting','on');
      | 
      |     % Connect "bitwise_or" to "delay"
      |     add_line(gcb, ['bitwise_or/1'], ['delay/1'],...
      |         'autorouting','on');
      | 
      |     % Connect "delay" to "multiport_switch"
      |     add_line(gcb, ['delay/1'], ['multiport_switch/1'],...
      |         'autorouting','on');
      | 
      |     % Connect "multiport_switch" to "rd_data"
      |     add_line(gcb, ['multiport_switch/1'], ['rd_data/1'],...
      |         'autorouting','on');
      |     
      | end
      | 
      | % If there is a half bram we must change a few parameters. Firstly, delete
      | % the write and read address lines. Then add bitslice blocks to reduce the
      | % address space in half. Connect rd_addr and wr_addr to the corresponding ports
      | % on the bram. Finally, change the address depth.
      | if halfbram
      |     
      |     if ceil(numbram) > 1
      |         
      |         % Delete lines
      |         delete_line(gcb, ['wr_address/1'], ['simple_ram_', int2str(i-1), '/2'])
      |         delete_line(gcb, ['rd_address/1'], ['simple_ram_', int2str(i-1), '/4'])
      |         
      |         % Write Address half ram Slice
      |         add_block('hdlsllib/Logic and Bit Operations/Bit Slice',...
      |                 [gcb, '/wr_address_hr'], 'Position',...
      |                 [160 130+(y-1)*600 250 170+(y-1)*600]);
      |         % Set bitslice parameters
      |         set_param([gcb, '/wr_address_hr'],...
      |             'lidx', int2str(log2(a(1))-2));
      |         set_param([gcb, '/wr_address_hr'],...
      |             'ridx', int2str(0));
      | 
      |         % Read Address half ram Slice
      |         add_block('hdlsllib/Logic and Bit Operations/Bit Slice',...
      |                 [gcb, '/rd_address_hr'], 'Position',...
      |                 [160 330+(y-1)*600 250 370+(y-1)*600]);
      |         % Set bitslice parameters
      |         set_param([gcb, '/rd_address_hr'],...
      |             'lidx', int2str(log2(a(1))-2));
      |         set_param([gcb, '/rd_address_hr'],...
      |             'ridx', int2str(0));
      | 
      |         % Connect "wr_addr" to "wr_address_hr"
      |         add_line(gcb, 'wr_addr/1', ['wr_address_hr', '/1'],...
      |             'autorouting','on');
      | 
      |         % Connect "rd_addr" to "rd_address_hr"
      |         add_line(gcb, 'rd_addr/1', ['rd_address_hr', '/1'],...
      |             'autorouting','on');
      | 
      |         % Connect "wr_address_hr" to "simple_ram_i"
      |         add_line(gcb, ['wr_address_hr', '/1'], ['simple_ram_', int2str(i-1), '/2'],...
      |             'autorouting','on');
      | 
      |         % Connect "rd_address_hr" to "simple_ram_i"
      |         add_line(gcb, ['rd_address_hr', '/1'], ['simple_ram_', int2str(i-1), '/4'],...
      |             'autorouting','on');
      |         
      |         % Update the ram parameters (address bits)
      |         set_param([gcb, '/simple_ram_', int2str(i-1)],...
      |             'ram_size', int2str(log2(a(1)/2)));
      | 
      |     else
      |         % Set bitslice parameters
      |         % set_param([gcb, '/wr_address'],...
      |         %     'lidx', int2str(log2(a(1))-2));
      |         % set_param([gcb, '/wr_address'],...
      |         %     'ridx', int2str(0));
      |         % Set bitslice parameters
      |         % set_param([gcb, '/rd_address'],...
      |         %     'lidx', int2str(log2(a(1))-2));
      |         % set_param([gcb, '/rd_address'],...
      |         %     'ridx', int2str(0));
      |         
      |     end
      |     
      | 
      |     
      | end
  RBM : Outport
  wires:
  simple_block_ram/1(rd_data) -> RBM/1
  Address/1 -> simple_block_ram/4(rd_addr), simple_block_ram/2(wr_addr)
  Enable/1 -> simple_block_ram/3(wr_en)
  Mode/1 -> simple_block_ram/1(wr_data)
